simulink model "pointmass_param_mpc"  (Simulink 8.3)
settings: Solver=ode4  StartTime=0.0  StopTime=200  RelTol=1e-3
undefined symbols (not defined in the file): A, B, bd, bx, C, dt, Ed, ef, Ef, Ef_block, f, ff, Fp, Fpf, Fps, fs, Fu, Fus, Fx, Fxf, Fxs, g, gt, H, hc, hcs, hp, hps, hx, hxs, P, Ps, q, Q, qf, Qf, R, r
libraries: simulink x1
settings Model: Creator=aeagr  LastModifiedBy=aeagr
settings OptimizationCC: ExpressionDepthLimit=2147483647
settings DebuggingCC: FcnCallInpInsideContextMsg=EnableAllAsWarning

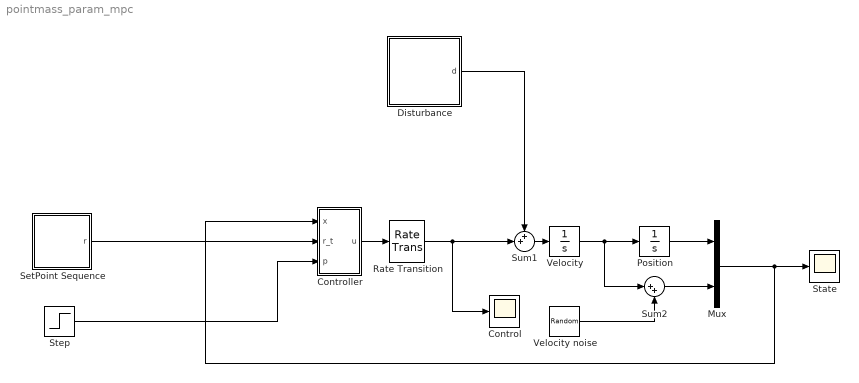
== system pointmass_param_mpc ==
  Control : Scope
      settings: TimeRange=240  YMin=-0.4  YMax=0.35
  Controller : Subsystem  TreatAsAtomicUnit=on  SystemSampleTime=dt
  Disturbance : Subsystem
  Mux : Mux  Inputs=2
  Position : Integrator
  Rate Transition : RateTransition
  SetPoint Sequence : Subsystem
  State : Scope
      settings: TimeRange=200  YMin=-1  YMax=14
  Step : Step  Time=100  Before=0.15  After=0  SampleTime=0
  Sum1 : Sum  Inputs=++|
  Sum2 : Sum  Inputs=|++
  Velocity : Integrator
  Velocity noise : RandomNumber  Variance=0.000000001  SampleTime=dt
  wires:
  Velocity/1 -> Position/1, Sum2/1
  Mux/1 -> Controller/1(x), State/1
  Position/1 -> Mux/1
  Sum1/1 -> Velocity/1
  Sum2/1 -> Mux/2
  Velocity noise/1 -> Sum2/2
  Disturbance/1(d) -> Sum1/1
  SetPoint Sequence/1(r) -> Controller/2(r_t)
  Step/1 -> Controller/3(p)
  Controller/1(u) -> Rate Transition/1
  Rate Transition/1 -> Control/1, Sum1/2

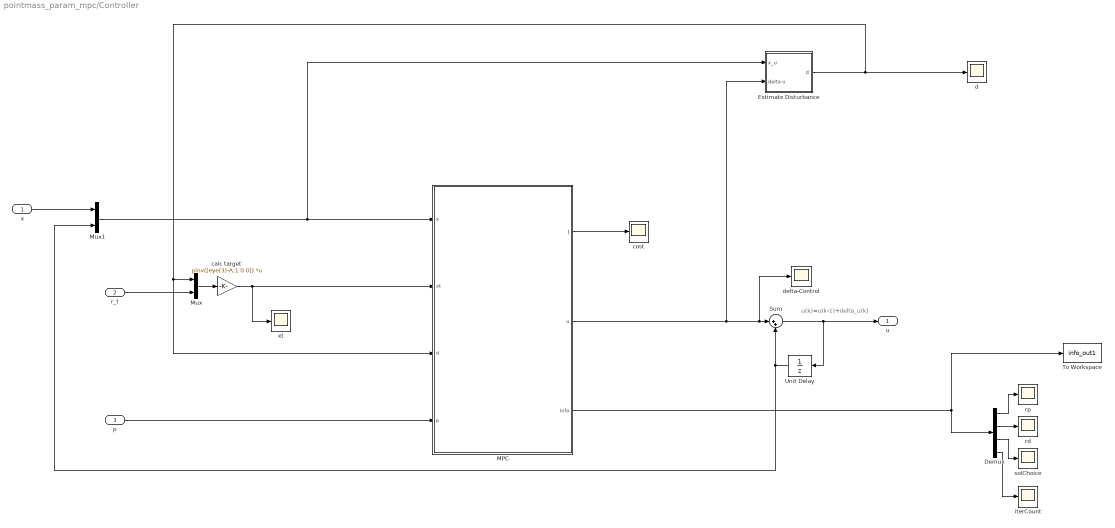
== system pointmass_param_mpc/Controller ==
  note: u(k)=u(k-1)+delta_u(k)
  x : Inport
  r_t : Inport  Port=2
  p : Inport  Port=3
  Demux : Demux
  Estimate Disturbance : Subsystem
  MPC : Subsystem  TreatAsAtomicUnit=on  mask{A=A, B=B, T=5, dt=-1, Q=Q, R=R, Qf=Qf, qv=q, rv=r, qfv=qf, Fx=Fx, Fu=Fu, Fp=Fp, f=f, Fxs=Fxs, Fus=Fus, Fps=Fps, fs=fs, Fxf=Fxf, Fpf=Fpf, ff=ff, Ef=Ef, Ed=Ed, e=ef, consAllBox=on, numNewton=5, kappa=0.005}
      mask prompts: T "Horizon length T"; dt "Time step"; qv "q"; rv "r"; qfv "qf"; e "ef"; consAllBox "Box constraints"; numNewton "Number of Newton Iterations"; kappa "Barrier weight kappa"
      mask init:
      | % build the big matrices
      | [H,g,gt,P,hx,hc,C,bx,bd,Ps,hxs,hcs,Ef_block,Ed_block,ef_block,hp,hps] = buildmatrices(A,B,Q,R,qv,rv,Qf,qfv,T,Fx,Fu,f,Fxs,Fus,fs,Fxf,ff,Ef,e,Ed,Fp,Fps,Fpf);
      | 
      | % options
      | opts=[];
      | disp(consAllBox)
      | if consAllBox,
      |     opts(1)=1; % 1 = assume diagonal Phi when solving
      | else
      |     opts(1)=0;
      | end
      | opts(2)=numNewton; % Newton iterations
      | opts(3)=1; % 1 = use soft constraints
      | opts(4)=0; % 1 = checking on
      | opts(7)=kappa; % tuning of barrier weight kappa
  Mux : Mux  Inputs=2
  Mux1 : Mux  Inputs=2
  Sum : Sum  Inputs=|++
  To Workspace : ToWorkspace  VariableName=info_out1  SampleTime=-1
  Unit Delay : UnitDelay  SampleTime=-1
  calc target : Gain  Gain=pinv([eye(3)-A;1 0 0])  Multiplication=Matrix(K*u)
  cost : Scope
      settings: YMin=-0.25  YMax=2.5  SaveName=ScopeData10
  d : Scope
      settings: YMin=-0.00025  YMax=0.002  SaveName=ScopeData11
  delta-Control : Scope
      settings: TimeRange=240  YMin=-0.4  YMax=0.35  SaveName=ScopeData2
  iterCount : Scope
      settings: TimeRange=200  YMin=0  YMax=25  SaveName=ScopeData12
  rd : Scope
      settings: YMin=0  YMax=13  SaveName=ScopeData13
  rp : Scope
      settings: YMin=1.65436e-24  YMax=2.75e-08  SaveName=ScopeData14
  solChoice : Scope
      settings: YMin=0.95  YMax=1.05  SaveName=ScopeData15
  xt : Scope
      settings: YMin=-0.25  YMax=2.5  SaveName=ScopeData16
  u : Outport
  wires:
  Sum/1 -> u/1, Unit Delay/1
  MPC/2(u) -> Sum/1, delta-Control/1, Estimate Disturbance/2(delta-u)
  Unit Delay/1 -> Sum/2, Mux1/2
  Mux1/1 -> MPC/1(x), Estimate Disturbance/1(x_u)
  Demux/1 -> rp/1
  Demux/2 -> rd/1
  Demux/3 -> solChoice/1
  Estimate Disturbance/1(d) -> MPC/3(d), Mux/1, d/1
  Mux/1 -> calc target/1
  r_t/1 -> Mux/2
  calc target/1 -> MPC/2(xt), xt/1
  Demux/4 -> iterCount/1
  MPC/3(info) -> To Workspace/1, Demux/1
  p/1 -> MPC/4(p)
  MPC/1(J) -> cost/1
  x/1 -> Mux1/1

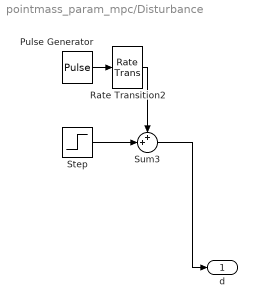
== system pointmass_param_mpc/Disturbance ==
  Pulse Generator : DiscretePulseGenerator  PulseType=Time based  Amplitude=0.1  Period=200  PhaseDelay=100
  Rate Transition2 : RateTransition
  Step : Step  Time=100  After=0.01  SampleTime=0
  Sum3 : Sum  Inputs=++|
  d : Outport
  wires:
  Step/1 -> Sum3/2
  Pulse Generator/1 -> Rate Transition2/1
  Sum3/1 -> d/1
  Rate Transition2/1 -> Sum3/1

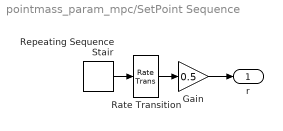
== system pointmass_param_mpc/SetPoint Sequence ==
  Gain : Gain  Gain=0.5
  Rate Transition : RateTransition
  Repeating Sequence Stair : simulink/Sources/Repeating Sequence Stair  OutValues=[1 0 2 0 3 0 4 0 5 0 6 0].'  tsamp=20  OutMin=[]  OutMax=[]  OutDataTypeStr=double  OutputDataTypeScalingMode=Specify via dialog  OutDataType=double  ConRadixGroup=Best Precision: Vector-wise  OutScaling=2^-12
  r : Outport
  wires:
  Repeating Sequence Stair/1 -> Rate Transition/1
  Rate Transition/1 -> Gain/1
  Gain/1 -> r/1

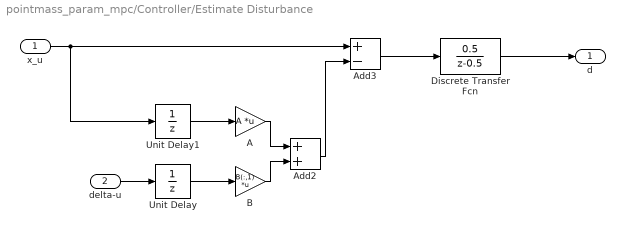
== system pointmass_param_mpc/Controller/Estimate Disturbance ==
  x_u : Inport
  delta-u : Inport  Port=2
  A : Gain  Gain=A  Multiplication=Matrix(K*u)
  Add2 : Sum
  Add3 : Sum  Inputs=+-
  B : Gain  Gain=B(:,1)  Multiplication=Matrix(K*u)
  Discrete Transfer Fcn : DiscreteTransferFcn  Numerator=[0.5]  Denominator=[1 -0.5]
  Unit Delay : UnitDelay  SampleTime=-1
  Unit Delay1 : UnitDelay  SampleTime=-1
  d : Outport
  wires:
  Unit Delay1/1 -> A/1
  Unit Delay/1 -> B/1
  A/1 -> Add2/1
  B/1 -> Add2/2
  Add2/1 -> Add3/2
  x_u/1 -> Unit Delay1/1, Add3/1
  delta-u/1 -> Unit Delay/1
  Add3/1 -> Discrete Transfer Fcn/1
  Discrete Transfer Fcn/1 -> d/1

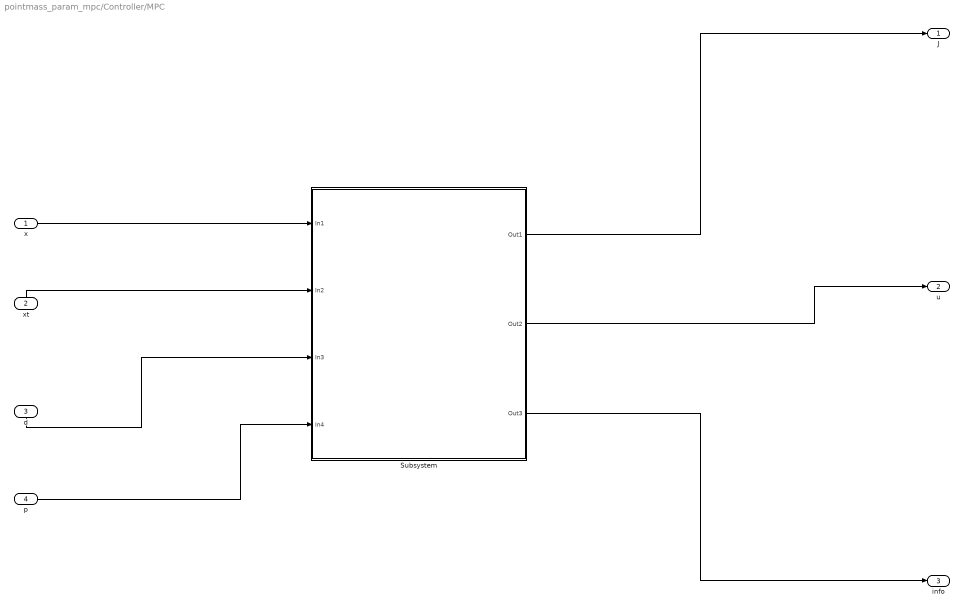
== system pointmass_param_mpc/Controller/MPC ==
  x : Inport
  xt : Inport  Port=2
  d : Inport  Port=3
  p : Inport  Port=4
  Subsystem : Subsystem  TreatAsAtomicUnit=on  SystemSampleTime=dt
  J : Outport
  u : Outport  Port=2
  info : Outport  Port=3
  wires:
  x/1 -> Subsystem/1(In1)
  xt/1 -> Subsystem/2(In2)
  d/1 -> Subsystem/3(In3)
  p/1 -> Subsystem/4(In4)
  Subsystem/1(Out1) -> J/1
  Subsystem/2(Out2) -> u/1
  Subsystem/3(Out3) -> info/1

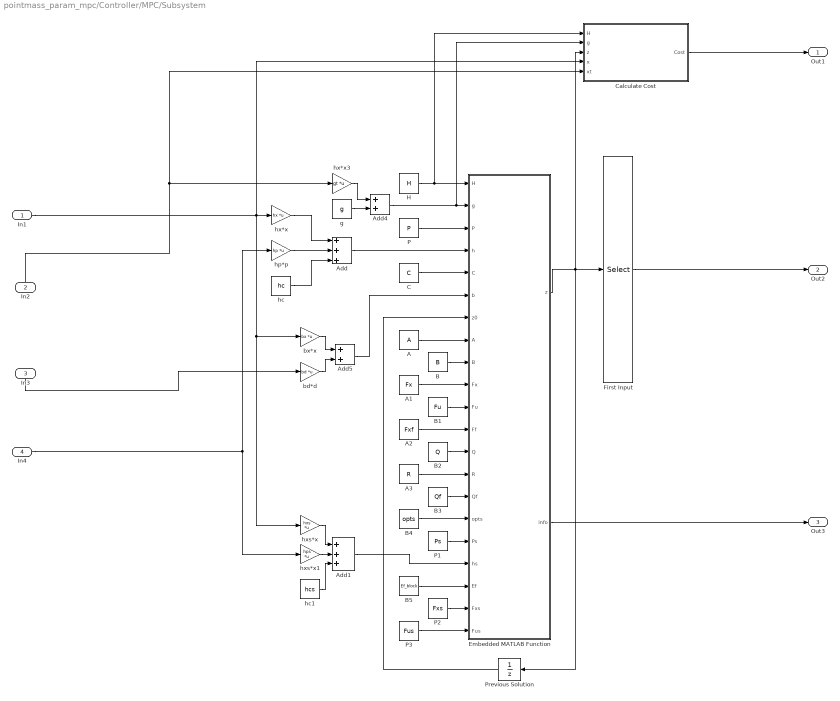
== system pointmass_param_mpc/Controller/MPC/Subsystem ==
  In1 : Inport
  In2 : Inport  Port=2
  In3 : Inport  Port=3
  In4 : Inport  Port=4
  A : Constant  Value=A
  A1 : Constant  Value=Fx
  A2 : Constant  Value=Fxf
  A3 : Constant  Value=R
  Add : Sum  Inputs=+++
  Add1 : Sum  Inputs=+++
  Add4 : Sum
  Add5 : Sum
  B : Constant  Value=B
  B1 : Constant  Value=Fu
  B2 : Constant  Value=Q
  B3 : Constant  Value=Qf
  B4 : Constant  Value=opts
  B5 : Constant  Value=Ef_block
  C : Constant  Value=C
  Calculate Cost : Subsystem
  Embedded MATLAB Function : MATLAB Function  TreatAsAtomicUnit=on
      settings: RTWFileNameOpts=Use subsystem name
  First Input : Selector  InputPortWidth=size(H,1)  Indices=1:size(B,2)
  H : Constant  Value=H
  P : Constant  Value=P
  P1 : Constant  Value=Ps
  P2 : Constant  Value=Fxs
  P3 : Constant  Value=Fus
  Previous Solution : UnitDelay  SampleTime=-1
  bd*d : Gain  Gain=bd  Multiplication=Matrix(K*u)
  bx*x : Gain  Gain=bx  Multiplication=Matrix(K*u)
  g : Constant  Value=g
  hc : Constant  Value=hc
  hc1 : Constant  Value=hcs
  hp*p : Gain  Gain=hp  Multiplication=Matrix(K*u)
  hx*x : Gain  Gain=hx  Multiplication=Matrix(K*u)
  hx*x3 : Gain  Gain=gt  Multiplication=Matrix(K*u)
  hxs*x : Gain  Gain=hxs  Multiplication=Matrix(K*u)
  hxs*x1 : Gain  Gain=hps  Multiplication=Matrix(K*u)
  Out1 : Outport
  Out2 : Outport  Port=2
  Out3 : Outport  Port=3
  wires:
  H/1 -> Embedded MATLAB Function/1(H), Calculate Cost/1(H)
  Embedded MATLAB Function/1(z) -> Previous Solution/1, First Input/1, Calculate Cost/3(z)
  Previous Solution/1 -> Embedded MATLAB Function/7(z0)
  B/1 -> Embedded MATLAB Function/9(B)
  hx*x/1 -> Add/1
  Add/1 -> Embedded MATLAB Function/4(h)
  A3/1 -> Embedded MATLAB Function/14(R)
  P/1 -> Embedded MATLAB Function/3(P)
  C/1 -> Embedded MATLAB Function/5(C)
  B3/1 -> Embedded MATLAB Function/15(Qf)
  A/1 -> Embedded MATLAB Function/8(A)
  First Input/1 -> Out2/1
  In2/1 -> Calculate Cost/5(xt), hx*x3/1
  In3/1 -> bd*d/1
  In1/1 -> Calculate Cost/4(x), bx*x/1, hxs*x/1, hx*x/1
  A2/1 -> Embedded MATLAB Function/12(Ff)
  g/1 -> Add4/2
  P2/1 -> Embedded MATLAB Function/20(Fxs)
  Embedded MATLAB Function/2(info) -> Out3/1
  In4/1 -> hp*p/1, hxs*x1/1
  Add1/1 -> Embedded MATLAB Function/18(hs)
  A1/1 -> Embedded MATLAB Function/10(Fx)
  bx*x/1 -> Add5/1
  hxs*x/1 -> Add1/1
  Add4/1 -> Embedded MATLAB Function/2(g), Calculate Cost/2(g)
  B1/1 -> Embedded MATLAB Function/11(Fu)
  hx*x3/1 -> Add4/1
  hp*p/1 -> Add/2
  hxs*x1/1 -> Add1/2
  hc1/1 -> Add1/3
  P3/1 -> Embedded MATLAB Function/21(Fus)
  B5/1 -> Embedded MATLAB Function/19(Ef)
  P1/1 -> Embedded MATLAB Function/17(Ps)
  hc/1 -> Add/3
  bd*d/1 -> Add5/2
  Add5/1 -> Embedded MATLAB Function/6(b)
  B4/1 -> Embedded MATLAB Function/16(opts)
  B2/1 -> Embedded MATLAB Function/13(Q)
  Calculate Cost/1(Cost) -> Out1/1

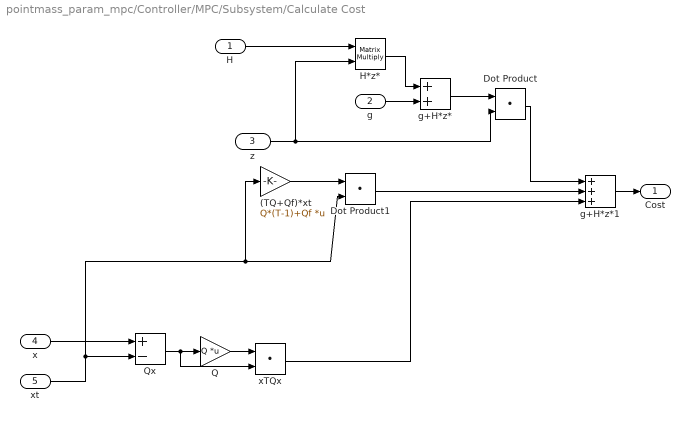
== system pointmass_param_mpc/Controller/MPC/Subsystem/Calculate Cost ==
  H : Inport
  g : Inport  Port=2
  z : Inport  Port=3
  x : Inport  Port=4
  xt : Inport  Port=5
  (TQ+Qf)*xt : Gain  Gain=Q*(T-1)+Qf  Multiplication=Matrix(K*u)
  Dot Product : DotProduct  InputSameDT=on  OutDataTypeStr=Inherit: Inherit via internal rule
  Dot Product1 : DotProduct  InputSameDT=on  OutDataTypeStr=Inherit: Inherit via internal rule
  H*z* : Product  Multiplication=Matrix(*)  RndMeth=Zero
  Q : Gain  Gain=Q  Multiplication=Matrix(K*u)
  Qx : Sum  Inputs=+-
  g+H*z* : Sum
  g+H*z*1 : Sum  Inputs=+++
  xTQx : DotProduct  InputSameDT=on  OutDataTypeStr=Inherit: Inherit via internal rule
  Cost : Outport
  wires:
  H*z*/1 -> g+H*z*/1
  g+H*z*/1 -> Dot Product/1
  (TQ+Qf)*xt/1 -> Dot Product1/1
  Dot Product/1 -> g+H*z*1/1
  Dot Product1/1 -> g+H*z*1/2
  Qx/1 -> Q/1, xTQx/2
  Q/1 -> xTQx/1
  xTQx/1 -> g+H*z*1/3
  H/1 -> H*z*/1
  g/1 -> g+H*z*/2
  z/1 -> H*z*/2, Dot Product/2
  x/1 -> Qx/1
  xt/1 -> Qx/2, (TQ+Qf)*xt/1, Dot Product1/2
  g+H*z*1/1 -> Cost/1

== matlab function Controller/MPC/Subsystem/Embedded MATLAB Function ==
  data: H input double; z output double; g input double; P input double; h input double; C input double; b input double size=size(C,1); z0 input double; A input double; B input double; Fx input double; Fu input double; Ff input double; Q input double; R input double; Qf input double; info output double; opts input double; Ps input double; hs input double; Ef input double; Fxs input double; Fus input double
function [z,info] = mpcsolve_simk(H,g,P,h,C,b,z0,A,B,Fx,Fu,Ff,Q,R,Qf,opts,Ps,hs,Ef,Fxs,Fus)
%#codegen

% just call to the Matlab version
[z,info] = mpcsolve(H,g,P,h,C,b,z0,A,B,Fx,Fu,Ff,Q,R,Qf,opts,Ps,hs,Ef,Fxs,Fus);
